simulink model "lab1"  (R2023a)
settings: Solver=VariableStepAuto  StartTime=0.0  StopTime=10  RelTol=1e-3
values from neighbouring files (symbols this model uses):
  C_m = 1.3    [untitled.m]
  C_w = 3.15    [untitled.m]
  J = 7*10^(-6)    (= 7e-06)    [untitled.m]
  L_a = 0.0015    [untitled.m]
  L_o = 0.013    [untitled.m]
  R = 8    [untitled.m]
settings Model: Creator=lizar  LastModifiedBy=diontep

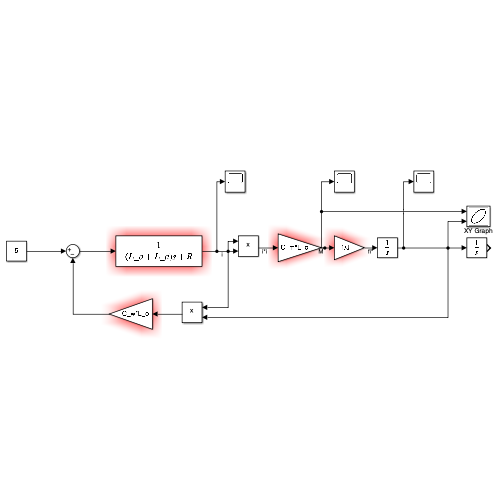
[thumbnail: Simulink's stored preview of the top-level diagram]
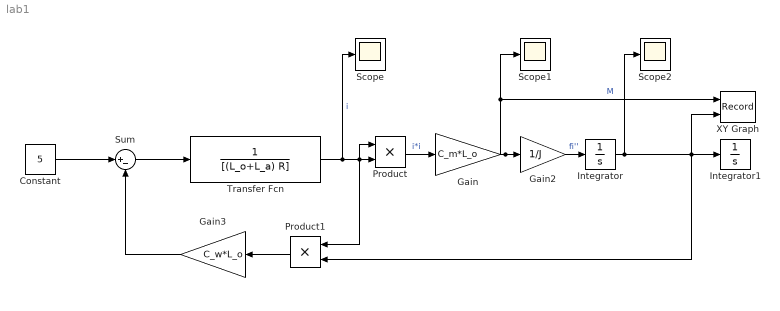
== system lab1 ==
  Constant : Constant  Value=5
  Gain : Gain  Gain=C_m*L_o
  Gain2 : Gain  Gain=1/J
  Gain3 : Gain  Gain=C_w*L_o
  Integrator : Integrator
  Integrator1 : Integrator
  Product : Product
  Product1 : Product
  Scope : Scope
  Scope1 : Scope
  Scope2 : Scope
  Sum : Sum  Inputs=|+-
  Transfer Fcn : TransferFcn  Denominator=[(L_o+L_a) R]
  XY Graph : Record  FileSettingsInternal="{\"entries\":[{\"content\":{\"excelSettings\":{\"content\":{},\"type\":\"Streamout.ExcelSettings\"}},\"type\":\"Streamout.FileSettingStorage\",\"uuid\":\"\"}],\"packageUris\":[\"http:\\/\\/schema.mathworks.com\\/mf0\\/streamout_blocks\\/R2020a\"],\"version\":\"1.0\"}"  Layout=[1 1]  SignalsInternal="{\"entries\":[{\"content\":{\"signals\":[{\"content\":{\"blockPath\":[],\"dimensions\":[1],\"domain\":\"\",\"lineColor\":\"#a2142f\",\"plots\":[1],\"port\":1,\"signalID\":8,\"signalName\":\"M\"},\"type\":\"RecordBlkView.Signal\",\"uuid\":\"\"},{\"content\":{\"blockPath\":[],\"dimensions\":[1],\"domain\":\"\",\"lineColor\":\"#139fff\",\"plots\":[1],\"port\":2,\"signalID\":11,\"signalName\":\"Integrator\"},\"type\":\"RecordBlkView.Signal\",\"uuid\":\"\"}]},\"type\":\"RecordBlkView.InputSignals\",\"uuid\":\"\"}],\"packageUris\":[\"http:\\/\\/schema.mathworks.com\\/mf0\\/streamout_blocks\\/R2020a\"],\"version\":\"1.0\"}"  VisualizationBindings="{\"xyplotplugin\":{\"info\":[{\"series\":[{\"bindingParametersList\":[{\"parameter\":\"X-Axis\",\"signalID\":8,\"signalName\":\"M\"},{\"parameter\":\"Y-Axis\",\"signalID\":11,\"signalName\":\"Integrator\"}],\"seriesID\":65209}],\"subplotID\":1}]}}"  CompatibilityTag=XY
  wires:
  Integrator/1 -> Scope2/1, Product1/2, XY Graph/2, Integrator1/1
  Sum/1 -> Transfer Fcn/1
  Transfer Fcn/1 -> Scope/1, Product/1, Product1/1, Product/2  "i"
  Product/1 -> Gain/1  "i*i"
  Gain/1 -> Scope1/1, XY Graph/1, Gain2/1  "M"
  Product1/1 -> Gain3/1
  Gain2/1 -> Integrator/1  "fi''"
  Gain3/1 -> Sum/2
  Constant/1 -> Sum/1
